simulink model "lab5_ASP_RyabchikvaM"  (R2022a)
settings: Solver=VariableStepAuto  StartTime=0.0  StopTime=10.0  RelTol=1e-3
libraries: dspsrcs4 x2, dspsnks4 x1, dspvision x1, dspfdesign x1
settings Model: Creator=masha  LastModifiedBy=masha

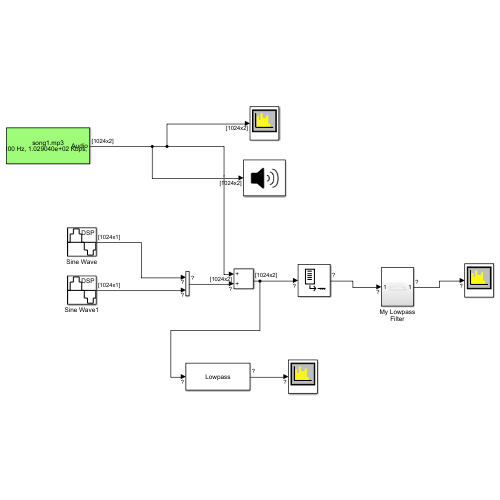
[thumbnail: Simulink's stored preview of the top-level diagram]
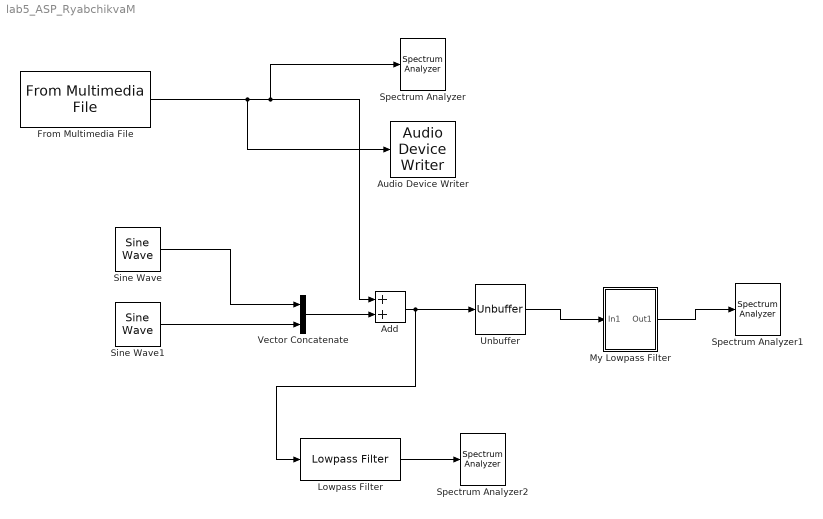
== system lab5_ASP_RyabchikvaM ==
  Add : Sum
  Audio Device Writer : dspsnks4/Audio Device Writer  Driver=DirectSound  Device=Default  InheritSampleRate=on  SampleRate=44100  BitDepth=16-bit integer  BufferSize=4096  NumBuffers=10  DefaultOutputChannelMapping=on  OutputChannelMapping=1:2  OutputNumUnderrunSamples=off  DriverIdx=1  DeviceWarnFlag=''
  From Multimedia File : dspvision/From Multimedia File  inputFilename=C:\Users\masha\Documents\MATLAB\song1.mp3  readRange=[1 Inf]  loop=on  numPlays=inf  outputStreams=Audio only  videoDataType=single  audioDataType=double  inheritSampleTime=on  userDefinedSampleTime=1/30  noAudioOutput=off  isIntensityVideo=off  fourcc=RGB  colorVideoFormat=Separate color signals  outputEOF=off  dataOrg=Column-major  audioFrameSize=1024  computeAudioFrameSize=off  outSamplingMode=Sample based
  Lowpass Filter : dspfdesign/Lowpass Filter  FilterType=FIR  DesignForMinimumOrder=on  FilterOrder=50  PassbandFrequency=8e3  StopbandFrequency=12e3  PassbandRipple=0.1  StopbandAttenuation=80  InheritSampleRate=off  SampleRate=44100  SimulateUsing=Interpreted execution  roundingMode=Floor  coeffsDataTypeStr=fixdt(1,16)
  My Lowpass Filter : Subsystem
  Sine Wave : dspsrcs4/Sine Wave  Amplitude=1  Frequency=17000  Phase=0  SampleMode=Discrete  OutComplex=Real  CompMethod=Trigonometric fcn  TableSize=Speed  SampleTime=1/44100  SamplesPerFrame=1024  ResetState=Restart at time zero  OutputFrames=off  dataType=double  wordLen=16  udDataType=sfix(16)  fracBitsMode=Best precision  numFracBits=15  OutDataTypeStr=double  LastOutDataTypeStr=double
  Sine Wave1 : dspsrcs4/Sine Wave  Amplitude=1  Frequency=17000  Phase=0  SampleMode=Discrete  OutComplex=Real  CompMethod=Trigonometric fcn  TableSize=Speed  SampleTime=1/44100  SamplesPerFrame=1024  ResetState=Restart at time zero  OutputFrames=off  dataType=double  wordLen=16  udDataType=sfix(16)  fracBitsMode=Best precision  numFracBits=15  OutDataTypeStr=double  LastOutDataTypeStr=double
  Spectrum Analyzer : SpectrumAnalyzer
  Spectrum Analyzer1 : SpectrumAnalyzer
  Spectrum Analyzer2 : SpectrumAnalyzer
  Unbuffer : Unbuffer
  Vector Concatenate : Concatenate  Mode=Multidimensional array  ConcatenateDimension=2
  wires:
  Sine Wave1/1 -> Vector Concatenate/2
  Vector Concatenate/1 -> Add/2
  From Multimedia File/1 -> Add/1, Spectrum Analyzer/1, Audio Device Writer/1
  Add/1 -> Lowpass Filter/1, Unbuffer/1
  My Lowpass Filter/1(Out1) -> Spectrum Analyzer1/1
  Lowpass Filter/1 -> Spectrum Analyzer2/1
  Unbuffer/1 -> My Lowpass Filter/1(In1)
  Sine Wave/1 -> Vector Concatenate/1

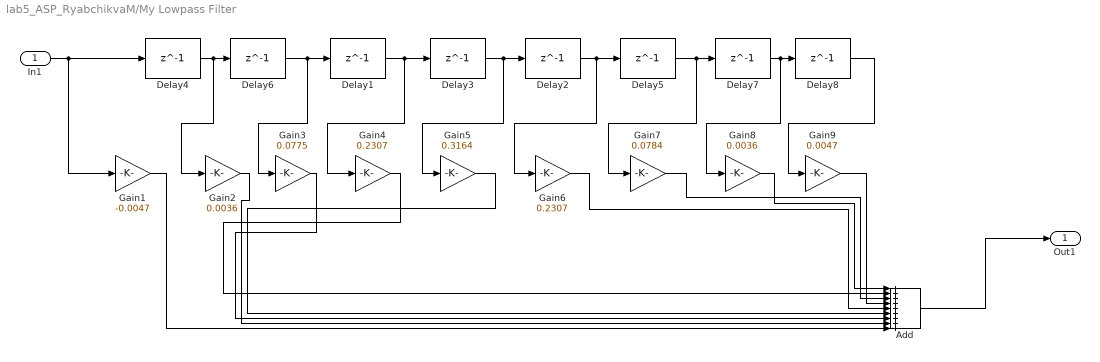
== system lab5_ASP_RyabchikvaM/My Lowpass Filter ==
  In1 : Inport
  Add : Sum  Inputs=+++++++++
  Delay{1..8} (8 alike) : Delay  DelayLength=1  InitialCondition=0  UseCircularBuffer=on
  Gain1 : Gain  Gain=-0.0047
  Gain2 : Gain  Gain=0.0036
  Gain3 : Gain  Gain=0.0775
  Gain4 : Gain  Gain=0.2307
  Gain5 : Gain  Gain=0.3164
  Gain6 : Gain  Gain=0.2307
  Gain7 : Gain  Gain=0.0784
  Gain8 : Gain  Gain=0.0036
  Gain9 : Gain  Gain=0.0047
  Out1 : Outport  VectorParamsAs1DForOutWhenUnconnected=off
  wires:
  Delay2/1 -> Gain6/1, Delay5/1
  Delay6/1 -> Gain3/1, Delay1/1
  Gain3/1 -> Add/7
  Delay7/1 -> Gain8/1, Delay8/1
  Delay5/1 -> Gain7/1, Delay7/1
  In1/1 -> Gain1/1, Delay4/1
  Gain4/1 -> Add/2
  Delay1/1 -> Gain4/1, Delay3/1
  Gain1/1 -> Add/9
  Add/1 -> Out1/1
  Delay4/1 -> Gain2/1, Delay6/1
  Delay8/1 -> Gain9/1
  Delay3/1 -> Gain5/1, Delay2/1
  Gain7/1 -> Add/3
  Gain6/1 -> Add/5
  Gain8/1 -> Add/1
  Gain5/1 -> Add/6
  Gain2/1 -> Add/8
  Gain9/1 -> Add/4
